simulink model "Q2part3"  (R2018b)
settings: Solver=VariableStepAuto  StartTime=0.0  StopTime=10.0  RelTol=1e-3
values from neighbouring files (symbols this model uses):
  A = [0           1                 0                          0 ... (first row only)    [Q2.m]
  B1 = [0 1/m1 0 1/m1+1/m2]'    [Q2.m]
  B2 = [0                 0 ... (first row only)    [Q2.m]
  C = [0 0 1 0]    [Q2.m]
  k1 = k(:,1:4)    [Q2.m]
  k2 = k(:,5)    [Q2.m]
settings Model: Creator=Asus  LastModifiedBy=Asus

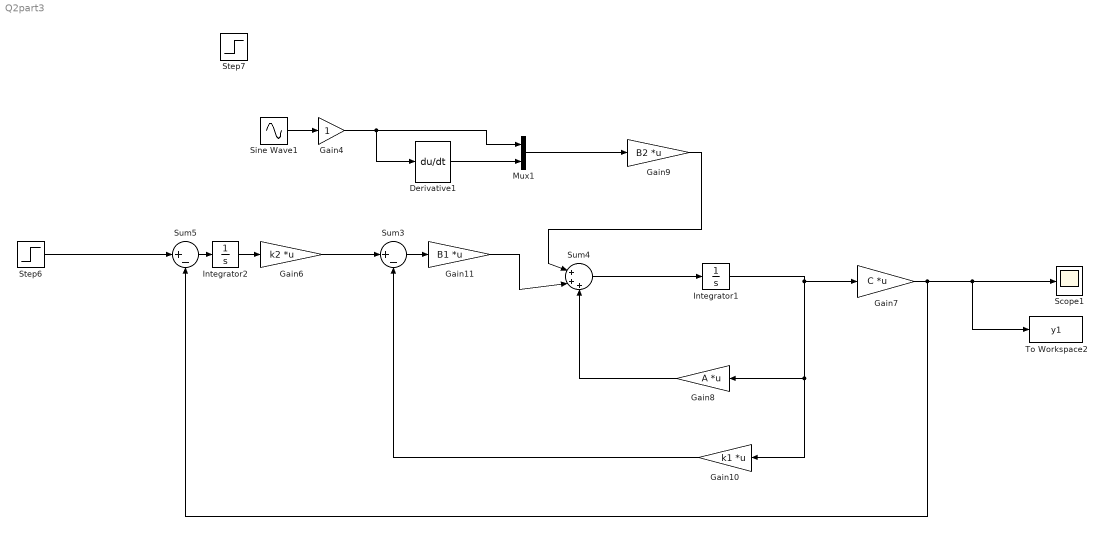
== system Q2part3 ==
  Derivative1 : Derivative
  Gain10 : Gain  Gain=k1  Multiplication=Matrix(K*u)
  Gain11 : Gain  Gain=B1  Multiplication=Matrix(K*u)
  Gain4 : Gain
  Gain6 : Gain  Gain=k2  Multiplication=Matrix(K*u)
  Gain7 : Gain  Gain=C  Multiplication=Matrix(K*u)
  Gain8 : Gain  Gain=A  Multiplication=Matrix(K*u)
  Gain9 : Gain  Gain=B2  Multiplication=Matrix(K*u)
  Integrator1 : Integrator
  Integrator2 : Integrator
  Mux1 : Mux  Inputs=2
  Scope1 : Scope
  Sine Wave1 : Sin  Amplitude=0.25  Frequency=2*pi  SampleTime=0
  Step6 : Step  Time=0  After=0  SampleTime=0
  Step7 : Step  Time=0  After=0.25  SampleTime=0
  Sum3 : Sum  Inputs=|+-
  Sum4 : Sum  Inputs=|+++
  Sum5 : Sum  Inputs=|+-
  To Workspace2 : ToWorkspace  VariableName=y1  SaveFormat=Timeseries  SampleTime=-1
  wires:
  Gain6/1 -> Sum3/1
  Sum3/1 -> Gain11/1
  Integrator1/1 -> Gain7/1, Gain8/1, Gain10/1
  Gain9/1 -> Sum4/1
  Sum4/1 -> Integrator1/1
  Gain10/1 -> Sum3/2
  Gain7/1 -> To Workspace2/1, Scope1/1, Sum5/2
  Gain4/1 -> Derivative1/1, Mux1/1
  Gain11/1 -> Sum4/2
  Sum5/1 -> Integrator2/1
  Integrator2/1 -> Gain6/1
  Derivative1/1 -> Mux1/2
  Gain8/1 -> Sum4/3
  Mux1/1 -> Gain9/1
  Step6/1 -> Sum5/1
  Sine Wave1/1 -> Gain4/1
